simulink model "DecentralizedPIControl"  (R2019a)
settings: Solver=VariableStepAuto  StartTime=0.0  StopTime=400  RelTol=1e-5
values from neighbouring files (symbols this model uses):
  Ao1 = pi * Do1^2 / 4    (= 0.17813934812)    [QuadrupleTank_SetUp.m]    (also in adeg_script.m)
  Ao2 = pi * Do2^2 / 4    (= 0.17813934812)    [QuadrupleTank_SetUp.m]    (also in adeg_script.m)
  Ao3 = pi * Do3^2 / 4    (= 0.17813934812)    [QuadrupleTank_SetUp.m]    (also in adeg_script.m)
  Ao4 = pi * Do4^2 / 4    (= 0.17813934812)    [QuadrupleTank_SetUp.m]    (also in adeg_script.m)
  At1 = pi * Dt1^2 / 4    (= 15.5179165474)    [QuadrupleTank_SetUp.m]    (also in adeg_script.m)
  At2 = pi * Dt2^2 / 4    (= 15.5179165474)    [QuadrupleTank_SetUp.m]    (also in adeg_script.m)
  At3 = pi * Dt3^2 / 4    (= 15.5179165474)    [QuadrupleTank_SetUp.m]    (also in adeg_script.m)
  At4 = pi * Dt4^2 / 4    (= 15.5179165474)    [QuadrupleTank_SetUp.m]    (also in adeg_script.m)
  g = 981    [QuadrupleTank_SetUp.m]    (also in adeg_script.m)
  gamma1 = Ai1/(Ai1+Ai4)    (= 0.64)    [QuadrupleTank_SetUp.m]    (also in adeg_script.m)
  gamma2 = Ai2/(Ai2+Ai3)    (= 0.64)    [QuadrupleTank_SetUp.m]    (also in adeg_script.m)
  Kl = 25/4.15    (= 6.02409638554)    [QuadrupleTank_SetUp.m]    (also in adeg_script.m)
  Kp = 1.289    [PI.m]    (also in QuadrupleTank_SetUp.m = 3.3; adeg_script.m = 3.3)
undefined symbols (not defined in the file or in its folder): lambda2
libraries: simulink x4
settings Model: Creator=adegbega  LastModifiedBy=hkhaj
settings DataIOCC: ReturnWorkspaceOutputs=off
settings DebuggingCC: ArithmeticOperatorsInVariantConditions=warning
settings SFSimCC: SimUseLocalCustomCode=off
settings RTWCC: RTWUseLocalCustomCode=off
settings CodeAppCC: StateflowObjectComments=on

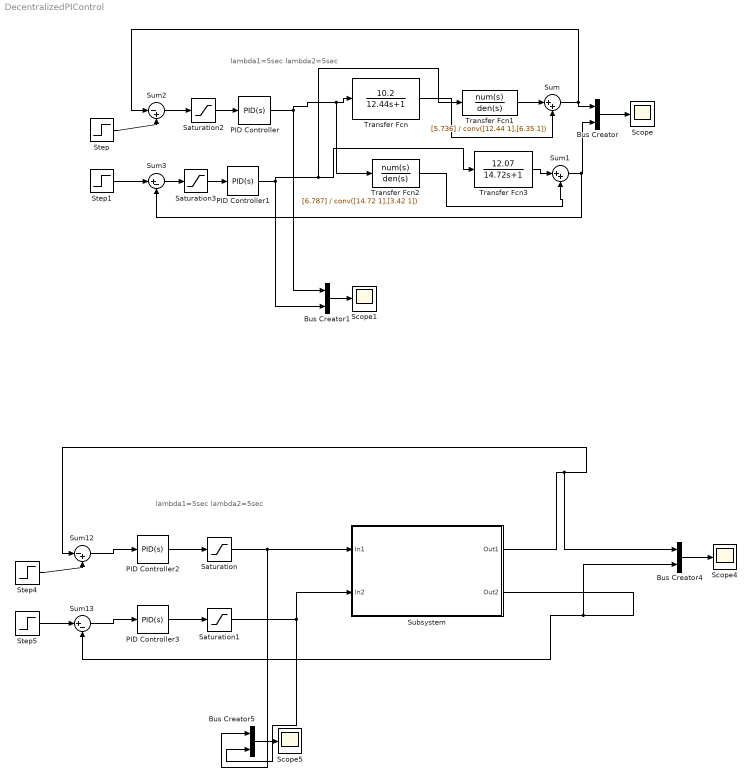
== system DecentralizedPIControl ==
  note: lambda1=5sec
      | lambda2=5sec
  note: lambda1=5sec
      | lambda2=5sec
  Bus Creator{,1,4..5} (4 alike) : BusCreator  Inputs=2
  PID Controller : simulink/Continuous/PID Controller  Controller=PID  Form=Parallel  TimeDomain=Continuous-time  SampleTime=-1  IntegratorMethod=Forward Euler  FilterMethod=Forward Euler  ControllerParametersSource=internal  P=1.2197/1  I=0.0981/1  D=0  UseFilter=on  N=100  TunerSelectOption=Transfer Function Based (PID Tuner App)  InitialConditionSource=internal  InitialConditionForIntegrator=0  InitialConditionForFilter=0  DifferentiatorICPrevScaledInput=0  ExternalReset=none  TrackingMode=off  Kt=1  LimitOutput=off  UpperSaturationLimit=inf  LowerSaturationLimit=-inf  LinearizeAsGain=on  AntiWindupMode=none  Kb=1  POutMin=[]  POutMax=[]  IOutMin=[]  IOutMax=[]  DOutMin=[]  DOutMax=[]  NOutMin=[]  NOutMax=[]  SumOutMin=[]  SumOutMax=[]  SaturationOutMin=[]  SaturationOutMax=[]  PParamMin=[]  PParamMax=[]  IParamMin=[]  IParamMax=[]  DParamMin=[]  DParamMax=[]  NParamMin=[]  NParamMax=[]  KbParamMin=[]  KbParamMax=[]  KtParamMin=[]  KtParamMax=[]  KbOutMin=[]  KbOutMax=[]  KtOutMin=[]  KtOutMax=[]  IntegratorOutMin=[]  IntegratorOutMax=[]  FilterOutMin=[]  FilterOutMax=[]  SumI1OutMin=[]  SumI1OutMax=[]  SumI2OutMin=[]  SumI2OutMax=[]  SumI3OutMin=[]  SumI3OutMax=[]  SumI4OutMin=[]  SumI4OutMax=[]  SumDOutMin=[]  SumDOutMax=[]  DifferentiatorOutMin=[]  DifferentiatorOutMax=[]  FilterDiffOutCoefMin=[]  FilterDiffOutCoefMax=[]  ReciprocalOutMin=[]  ReciprocalOutMax=[]  SumDenOutMin=[]  SumDenOutMax=[]  SumNumOutMin=[]  SumNumOutMax=[]  DivideOutMin=[]  DivideOutMax=[]  IntegratorContinuousStateAttributes=''  IntegratorStateMustResolveToSignalObject=off  IntegratorRTWStateStorageClass=Auto  FilterContinuousStateAttributes=''  FilterStateMustResolveToSignalObject=off  FilterRTWStateStorageClass=Auto  ParallelPVariant=InternalParameters  IdealPVariant=Disabled  IVariant=InternalParameters  DVariant=InternalParameters  IntegratorVariant=Continuous  SatVariant=Disabled  AWVariant=Passthrough  PCopyVariant=Disabled  TRVariant=Disabled  FdbkBlocksVariant=Forward  IdealPFdbkVariant=Disabled  SatFdbkVariant=Disabled  DerivativeFilterVariant=ContFilter  NVariant=InternalParameters  NCopyVariant=Disabled  FilterICVariant=InternalICsFilter  IntegratorICVariant=InternalICs  ExternalResetVariant=Disabled  TRSumVariant=Passthrough  SumFdbkVariant=Disabled  SumVariant=Sum_PID
  PID Controller1 : simulink/Continuous/PID Controller  Controller=PID  Form=Parallel  TimeDomain=Continuous-time  SampleTime=-1  IntegratorMethod=Forward Euler  FilterMethod=Forward Euler  ControllerParametersSource=internal  P=1.2197/1  I=0.0829/1  D=0  UseFilter=on  N=100  TunerSelectOption=Transfer Function Based (PID Tuner App)  InitialConditionSource=internal  InitialConditionForIntegrator=0  InitialConditionForFilter=0  DifferentiatorICPrevScaledInput=0  ExternalReset=none  TrackingMode=off  Kt=1  LimitOutput=off  UpperSaturationLimit=inf  LowerSaturationLimit=-inf  LinearizeAsGain=on  AntiWindupMode=none  Kb=1  POutMin=[]  POutMax=[]  IOutMin=[]  IOutMax=[]  DOutMin=[]  DOutMax=[]  NOutMin=[]  NOutMax=[]  SumOutMin=[]  SumOutMax=[]  SaturationOutMin=[]  SaturationOutMax=[]  PParamMin=[]  PParamMax=[]  IParamMin=[]  IParamMax=[]  DParamMin=[]  DParamMax=[]  NParamMin=[]  NParamMax=[]  KbParamMin=[]  KbParamMax=[]  KtParamMin=[]  KtParamMax=[]  KbOutMin=[]  KbOutMax=[]  KtOutMin=[]  KtOutMax=[]  IntegratorOutMin=[]  IntegratorOutMax=[]  FilterOutMin=[]  FilterOutMax=[]  SumI1OutMin=[]  SumI1OutMax=[]  SumI2OutMin=[]  SumI2OutMax=[]  SumI3OutMin=[]  SumI3OutMax=[]  SumI4OutMin=[]  SumI4OutMax=[]  SumDOutMin=[]  SumDOutMax=[]  DifferentiatorOutMin=[]  DifferentiatorOutMax=[]  FilterDiffOutCoefMin=[]  FilterDiffOutCoefMax=[]  ReciprocalOutMin=[]  ReciprocalOutMax=[]  SumDenOutMin=[]  SumDenOutMax=[]  SumNumOutMin=[]  SumNumOutMax=[]  DivideOutMin=[]  DivideOutMax=[]  IntegratorContinuousStateAttributes=''  IntegratorStateMustResolveToSignalObject=off  IntegratorRTWStateStorageClass=Auto  FilterContinuousStateAttributes=''  FilterStateMustResolveToSignalObject=off  FilterRTWStateStorageClass=Auto  ParallelPVariant=InternalParameters  IdealPVariant=Disabled  IVariant=InternalParameters  DVariant=InternalParameters  IntegratorVariant=Continuous  SatVariant=Disabled  AWVariant=Passthrough  PCopyVariant=Disabled  TRVariant=Disabled  FdbkBlocksVariant=Forward  IdealPFdbkVariant=Disabled  SatFdbkVariant=Disabled  DerivativeFilterVariant=ContFilter  NVariant=InternalParameters  NCopyVariant=Disabled  FilterICVariant=InternalICsFilter  IntegratorICVariant=InternalICs  ExternalResetVariant=Disabled  TRSumVariant=Passthrough  SumFdbkVariant=Disabled  SumVariant=Sum_PID
  PID Controller2 : simulink/Continuous/PID Controller  Controller=PID  Form=Parallel  TimeDomain=Continuous-time  SampleTime=-1  IntegratorMethod=Forward Euler  FilterMethod=Forward Euler  ControllerParametersSource=internal  P=1.2197/1  I=0.0981/1  D=0  UseFilter=on  N=100  TunerSelectOption=Transfer Function Based (PID Tuner App)  InitialConditionSource=internal  InitialConditionForIntegrator=0  InitialConditionForFilter=0  DifferentiatorICPrevScaledInput=0  ExternalReset=none  TrackingMode=off  Kt=1  LimitOutput=off  UpperSaturationLimit=inf  LowerSaturationLimit=-inf  LinearizeAsGain=on  AntiWindupMode=none  Kb=1  POutMin=[]  POutMax=[]  IOutMin=[]  IOutMax=[]  DOutMin=[]  DOutMax=[]  NOutMin=[]  NOutMax=[]  SumOutMin=[]  SumOutMax=[]  SaturationOutMin=[]  SaturationOutMax=[]  PParamMin=[]  PParamMax=[]  IParamMin=[]  IParamMax=[]  DParamMin=[]  DParamMax=[]  NParamMin=[]  NParamMax=[]  KbParamMin=[]  KbParamMax=[]  KtParamMin=[]  KtParamMax=[]  KbOutMin=[]  KbOutMax=[]  KtOutMin=[]  KtOutMax=[]  IntegratorOutMin=[]  IntegratorOutMax=[]  FilterOutMin=[]  FilterOutMax=[]  SumI1OutMin=[]  SumI1OutMax=[]  SumI2OutMin=[]  SumI2OutMax=[]  SumI3OutMin=[]  SumI3OutMax=[]  SumI4OutMin=[]  SumI4OutMax=[]  SumDOutMin=[]  SumDOutMax=[]  DifferentiatorOutMin=[]  DifferentiatorOutMax=[]  FilterDiffOutCoefMin=[]  FilterDiffOutCoefMax=[]  ReciprocalOutMin=[]  ReciprocalOutMax=[]  SumDenOutMin=[]  SumDenOutMax=[]  SumNumOutMin=[]  SumNumOutMax=[]  DivideOutMin=[]  DivideOutMax=[]  IntegratorContinuousStateAttributes=''  IntegratorStateMustResolveToSignalObject=off  IntegratorRTWStateStorageClass=Auto  FilterContinuousStateAttributes=''  FilterStateMustResolveToSignalObject=off  FilterRTWStateStorageClass=Auto  ParallelPVariant=InternalParameters  IdealPVariant=Disabled  IVariant=InternalParameters  DVariant=InternalParameters  IntegratorVariant=Continuous  SatVariant=Disabled  AWVariant=Passthrough  PCopyVariant=Disabled  TRVariant=Disabled  FdbkBlocksVariant=Forward  IdealPFdbkVariant=Disabled  SatFdbkVariant=Disabled  DerivativeFilterVariant=ContFilter  NVariant=InternalParameters  NCopyVariant=Disabled  FilterICVariant=InternalICsFilter  IntegratorICVariant=InternalICs  ExternalResetVariant=Disabled  TRSumVariant=Passthrough  SumFdbkVariant=Disabled  SumVariant=Sum_PID
  PID Controller3 : simulink/Continuous/PID Controller  Controller=PID  Form=Parallel  TimeDomain=Continuous-time  SampleTime=-1  IntegratorMethod=Forward Euler  FilterMethod=Forward Euler  ControllerParametersSource=internal  P=1.2197/lambda2  I=0.0829/lambda2  D=0  UseFilter=on  N=100  TunerSelectOption=Transfer Function Based (PID Tuner App)  InitialConditionSource=internal  InitialConditionForIntegrator=0  InitialConditionForFilter=0  DifferentiatorICPrevScaledInput=0  ExternalReset=none  TrackingMode=off  Kt=1  LimitOutput=off  UpperSaturationLimit=inf  LowerSaturationLimit=-inf  LinearizeAsGain=on  AntiWindupMode=none  Kb=1  POutMin=[]  POutMax=[]  IOutMin=[]  IOutMax=[]  DOutMin=[]  DOutMax=[]  NOutMin=[]  NOutMax=[]  SumOutMin=[]  SumOutMax=[]  SaturationOutMin=[]  SaturationOutMax=[]  PParamMin=[]  PParamMax=[]  IParamMin=[]  IParamMax=[]  DParamMin=[]  DParamMax=[]  NParamMin=[]  NParamMax=[]  KbParamMin=[]  KbParamMax=[]  KtParamMin=[]  KtParamMax=[]  KbOutMin=[]  KbOutMax=[]  KtOutMin=[]  KtOutMax=[]  IntegratorOutMin=[]  IntegratorOutMax=[]  FilterOutMin=[]  FilterOutMax=[]  SumI1OutMin=[]  SumI1OutMax=[]  SumI2OutMin=[]  SumI2OutMax=[]  SumI3OutMin=[]  SumI3OutMax=[]  SumI4OutMin=[]  SumI4OutMax=[]  SumDOutMin=[]  SumDOutMax=[]  DifferentiatorOutMin=[]  DifferentiatorOutMax=[]  FilterDiffOutCoefMin=[]  FilterDiffOutCoefMax=[]  ReciprocalOutMin=[]  ReciprocalOutMax=[]  SumDenOutMin=[]  SumDenOutMax=[]  SumNumOutMin=[]  SumNumOutMax=[]  DivideOutMin=[]  DivideOutMax=[]  IntegratorContinuousStateAttributes=''  IntegratorStateMustResolveToSignalObject=off  IntegratorRTWStateStorageClass=Auto  FilterContinuousStateAttributes=''  FilterStateMustResolveToSignalObject=off  FilterRTWStateStorageClass=Auto  ParallelPVariant=InternalParameters  IdealPVariant=Disabled  IVariant=InternalParameters  DVariant=InternalParameters  IntegratorVariant=Continuous  SatVariant=Disabled  AWVariant=Passthrough  PCopyVariant=Disabled  TRVariant=Disabled  FdbkBlocksVariant=Forward  IdealPFdbkVariant=Disabled  SatFdbkVariant=Disabled  DerivativeFilterVariant=ContFilter  NVariant=InternalParameters  NCopyVariant=Disabled  FilterICVariant=InternalICsFilter  IntegratorICVariant=InternalICs  ExternalResetVariant=Disabled  TRSumVariant=Passthrough  SumFdbkVariant=Disabled  SumVariant=Sum_PID
  Saturation : Saturate  UpperLimit=22  LowerLimit=0
  Saturation1 : Saturate  UpperLimit=22  LowerLimit=0
  Saturation2 : Saturate  UpperLimit=3  LowerLimit=-3
  Saturation3 : Saturate  UpperLimit=3  LowerLimit=-3
  Scope{,1,4..5} (4 alike) : Scope
  Step : Step  Time=150  After=15  SampleTime=0
  Step1 : Step  Time=0  After=20  SampleTime=0
  Step4 : Step  Time=150  After=15  SampleTime=0
  Step5 : Step  Time=0  After=20  SampleTime=0
  Subsystem : Subsystem
  Sum : Sum  Inputs=|++
  Sum1 : Sum  Inputs=|++
  Sum12 : Sum  Inputs=|-+
  Sum13 : Sum  Inputs=|+-
  Sum2 : Sum  Inputs=|-+
  Sum3 : Sum  Inputs=|+-
  Transfer Fcn : TransferFcn  Numerator=[10.2]  Denominator=[12.44 1]
  Transfer Fcn1 : TransferFcn  Numerator=[5.736]  Denominator=conv([12.44 1],[6.35 1])
  Transfer Fcn2 : TransferFcn  Numerator=[6.787]  Denominator=conv([14.72 1],[3.42 1])
  Transfer Fcn3 : TransferFcn  Numerator=[12.07]  Denominator=[14.72 1]
  wires:
  Transfer Fcn1/1 -> Sum/1
  Transfer Fcn/1 -> Sum/2
  Transfer Fcn2/1 -> Sum1/2
  Transfer Fcn3/1 -> Sum1/1
  Bus Creator/1 -> Scope/1
  PID Controller/1 -> Transfer Fcn/1, Transfer Fcn2/1, Bus Creator1/1
  PID Controller1/1 -> Transfer Fcn1/1, Transfer Fcn3/1, Bus Creator1/2
  Sum/1 -> Sum2/1, Bus Creator/1
  Sum1/1 -> Sum3/2, Bus Creator/2
  Step/1 -> Sum2/2
  Step1/1 -> Sum3/1
  Sum3/1 -> Saturation3/1
  Sum2/1 -> Saturation2/1
  Bus Creator1/1 -> Scope1/1
  Bus Creator5/1 -> Scope5/1
  Sum13/1 -> PID Controller3/1
  Sum12/1 -> PID Controller2/1
  Bus Creator4/1 -> Scope4/1
  Step5/1 -> Sum13/1
  Step4/1 -> Sum12/2
  PID Controller3/1 -> Saturation1/1
  PID Controller2/1 -> Saturation/1
  Subsystem/1(Out1) -> Sum12/1, Bus Creator4/1
  Subsystem/2(Out2) -> Sum13/2, Bus Creator4/2
  Saturation/1 -> Bus Creator5/1, Subsystem/1(In1)
  Saturation1/1 -> Subsystem/2(In2), Bus Creator5/2
  Saturation2/1 -> PID Controller/1
  Saturation3/1 -> PID Controller1/1

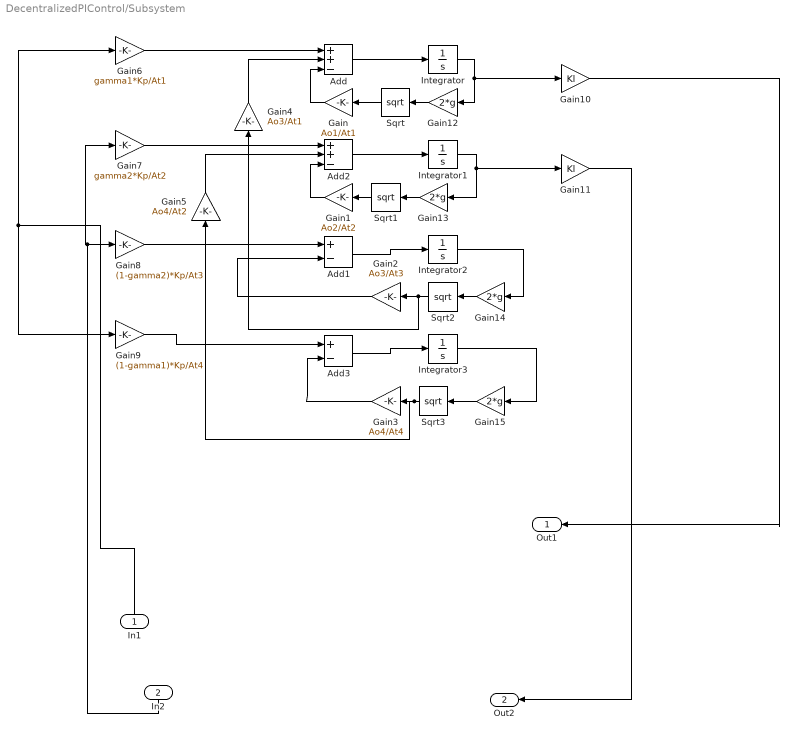
== system DecentralizedPIControl/Subsystem ==
  In1 : Inport
  In2 : Inport  Port=2
  Add : Sum  Inputs=++-
  Add1 : Sum  Inputs=+-
  Add2 : Sum  Inputs=++-
  Add3 : Sum  Inputs=+-
  Gain : Gain  Gain=Ao1/At1
  Gain1 : Gain  Gain=Ao2/At2
  Gain10 : Gain  Gain=Kl
  Gain11 : Gain  Gain=Kl
  Gain{12..15} (4 alike) : Gain  Gain=2*g
  Gain2 : Gain  Gain=Ao3/At3
  Gain3 : Gain  Gain=Ao4/At4
  Gain4 : Gain  Gain=Ao3/At1
  Gain5 : Gain  Gain=Ao4/At2
  Gain6 : Gain  Gain=gamma1*Kp/At1
  Gain7 : Gain  Gain=gamma2*Kp/At2
  Gain8 : Gain  Gain=(1-gamma2)*Kp/At3
  Gain9 : Gain  Gain=(1-gamma1)*Kp/At4
  Integrator{,1..3} (4 alike) : Integrator
  Sqrt : Sqrt  SaturateOnIntegerOverflow=on
  Sqrt1 : Sqrt  OutputSignalType=real  SaturateOnIntegerOverflow=on
  Sqrt2 : Sqrt  OutputSignalType=real  SaturateOnIntegerOverflow=on
  Sqrt3 : Sqrt  OutputSignalType=real  SaturateOnIntegerOverflow=on
  Out1 : Outport
  Out2 : Outport  Port=2
  wires:
  Sqrt2/1 -> Gain4/1, Gain2/1
  Gain9/1 -> Add3/1
  Add2/1 -> Integrator1/1
  Gain5/1 -> Add2/2
  Sqrt3/1 -> Gain5/1, Gain3/1
  Gain/1 -> Add/3
  Sqrt/1 -> Gain/1
  Gain6/1 -> Add/1
  Add3/1 -> Integrator3/1
  Gain7/1 -> Add2/1
  Gain8/1 -> Add1/1
  Sqrt1/1 -> Gain1/1
  Add/1 -> Integrator/1
  Gain1/1 -> Add2/3
  Gain3/1 -> Add3/2
  Integrator1/1 -> Gain13/1, Gain11/1
  Integrator2/1 -> Gain14/1
  Gain2/1 -> Add1/2
  Integrator/1 -> Gain12/1, Gain10/1
  Gain4/1 -> Add/2
  Add1/1 -> Integrator2/1
  Integrator3/1 -> Gain15/1
  Gain10/1 -> Out1/1
  Gain11/1 -> Out2/1
  Gain12/1 -> Sqrt/1
  Gain13/1 -> Sqrt1/1
  Gain14/1 -> Sqrt2/1
  Gain15/1 -> Sqrt3/1
  In1/1 -> Gain6/1, Gain9/1
  In2/1 -> Gain7/1, Gain8/1
